simulink model "RoombaLibraries"  (R2017b)
settings: Solver=VariableStepAuto  StartTime=0.0  StopTime=10.0  RelTol=1e-3
settings Model: Creator=segadiallo  LastModifiedBy=segadiallo

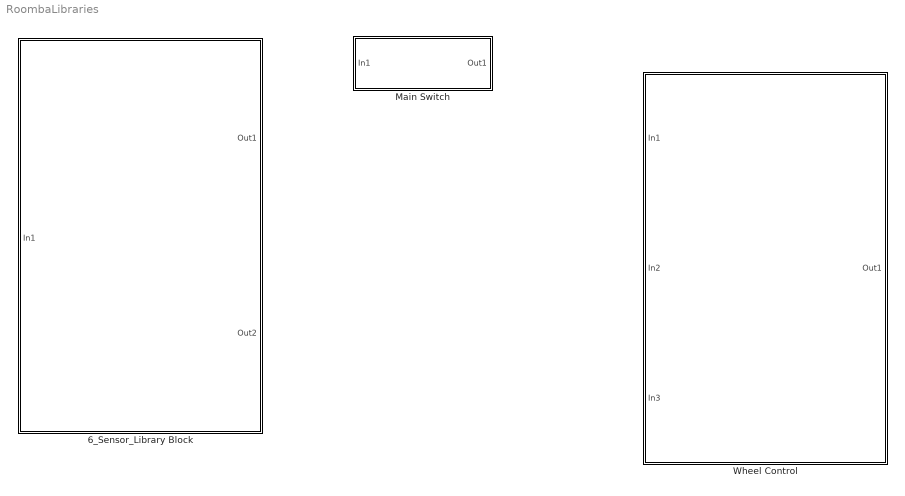
== system RoombaLibraries ==
  6_Sensor_Library Block : Subsystem
      mask help: IR Sensor Test
      mask Display:
      | disp('6_Sensors_Test')
      | port_label('output',1,'Status')
      | port_label('output',2,'display')
      | port_label('input',1,'InputV')
  Main Switch : Subsystem
      mask help: Main Switch
      mask Display:
      | disp('Main Switch')
      | port_label('output',1,'inputV')
      | port_label('input',1,'Go')
  Wheel Control : Subsystem
      mask help: Wheel Control
      mask Display:
      | disp('Wheel Controle');
      | port_label('output',1,'Status');
      | port_label('input',2,'rightW');
      | port_label('input',1,'InputV');
      | port_label('input',3,'leftW');

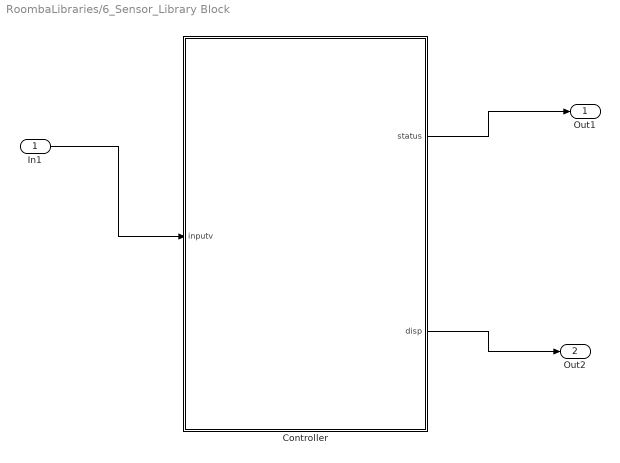
== system RoombaLibraries/6_Sensor_Library Block ==
  In1 : Inport
  Controller : Stateflow chart  TreatAsAtomicUnit=on
  Out1 : Outport
  Out2 : Outport  Port=2
  wires:
  Controller/2(disp) -> Out2/1
  Controller/1(status) -> Out1/1
  In1/1 -> Controller/1(inputv)

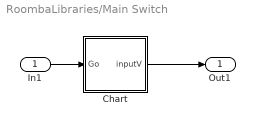
== system RoombaLibraries/Main Switch ==
  In1 : Inport
  Chart : Stateflow chart  TreatAsAtomicUnit=on
  Out1 : Outport
  wires:
  In1/1 -> Chart/1(Go)
  Chart/1(inputV) -> Out1/1

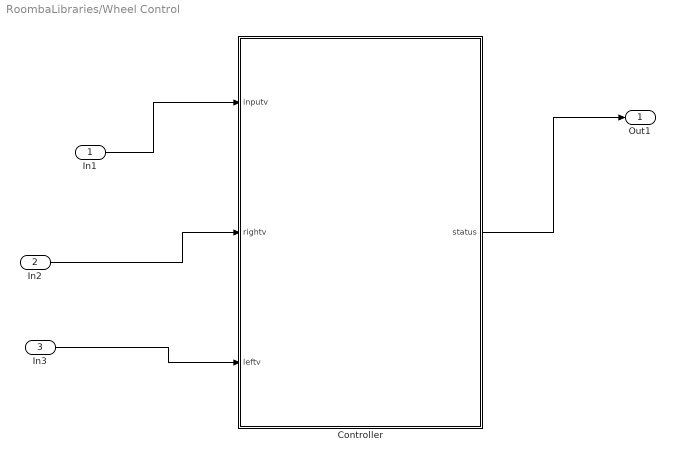
== system RoombaLibraries/Wheel Control ==
  In1 : Inport
  In2 : Inport  Port=2
  In3 : Inport  Port=3
  Controller : Stateflow chart  TreatAsAtomicUnit=on
  Out1 : Outport
  wires:
  In1/1 -> Controller/1(inputv)
  In2/1 -> Controller/2(rightv)
  In3/1 -> Controller/3(leftv)
  Controller/1(status) -> Out1/1

== stateflow chart RoombaLibraries/6_Sensor_Library Block/Controller ==
  state init
    entry:
    coder.extrinsic('evalin');
    obj = evalin('base','objWs');
    disp=[0;0;0;0;0;0];
    status = 0
  state NoCommand
    entry:
    disp=[0;0;0;0;0;0];
    status=0
  state Start
    entry:
    du:
    coder.extrinsic('evalin');
    obj = evalin('base','objWs');
    coder.extrinsic('RangeStateRoomba')
    disp=RangeStateRoomba(obj);
    status = 1;
  (default) -> NoCommand
  NoCommand -> init : after(0.5,sec)
  init -> Start : [inputv==3]
  Start -> init [order 2] : [inputv==1]
  Start -> Start [order 1] : after(0.1,sec)
  data: inputv input size=1; status output; so local; disp output double size=6; obj local

== stateflow chart RoombaLibraries/Wheel Control/Controller ==
  state NoCommand
    entry:
    status=0
  state Start
    during:
    entry:
    coder.extrinsic('evalin');
    obj = evalin('base','objWs');
    SetWheelVelRoomba(obj, rightv, leftv)
    status = 1;
  state Reset
    entry:
    coder.extrinsic('evalin');
    obj = evalin('base','objWs');
    fwrite(obj, 7)
  (default) -> NoCommand
  NoCommand -> Start : [inputv==3 ]
  Start -> Start [order 2] : after(0.1,sec)
  Start -> Reset [order 1] : [inputv==1]
  data: inputv input size=1; status output; so local; rightv input; leftv input

== stateflow chart RoombaLibraries/Main Switch/Chart ==
  state START
    entry:
    y=0
  state CONNECT
    entry: tcpInit;
  state DISCONNECT
    entry: y=0
    coder.extrinsic('evalin')
    obj=evalin('base','objWs')
    fclose(obj)
  state Toggle
    entry: y = y + 1
    if y==3
    y=1
    end
  state SerialControl1
    entry: y==1
  (default) -> START
  START -> CONNECT : [n==1]
  DISCONNECT -> CONNECT : [n==1]
  CONNECT -> DISCONNECT [order 1] : [n==0]
  SerialControl1 -> DISCONNECT [order 2] : [n==0]
  CONNECT -> SerialControl1 [order 2]
  Toggle -> SerialControl1 : after(1,sec)
  SerialControl1 -> Toggle [order 1] : [n==1]
  data: Go input; inputV output
  function tcpInit:
    | function tcpInit
    | coder.extrinsic('tcpip');
    | coder.extrinsic('assignin');
    | persistent obj
    | if isempty(obj)
    |     obj=tcpip('10.0.0.1',9001);
    |     assignin('base','objWs',obj);
    |  
    |     set(obj,'Terminator','LF');
    | set(obj,'InputBufferSize',1000)
    | set(obj, 'Timeout', .5)
    | set(obj, 'ByteOrder','bigEndian');
    | 
    |  
    |  fopen(obj);
    |  
    |  fwrite(obj,128);
    | pause(.1)
    | 
    | fwrite(obj,132);
    | pause(.1)
    | 
    | % %Print 'go' on display
    | fwrite(obj, [164, 71, 79, 32, 32]);
    | % make a sound
    | fwrite(obj, [140 1 3 60 20 72 20 84 40 ]); %RoombaInit Song
    | fwrite(obj, [140 2 1 60 20]); % BeepRoomba song
    | fwrite(obj, [140 3 3 84 20 72 30 60 40]); % PowerOffRoomba song
    | fwrite(obj, [141 1]); % play RoombaInit song
    | pause(1);
    | so=obj;
    | end
